simulink subsystem "PieroMMG"  (R2023b)
settings: Solver=VariableStepAuto  StartTime=0.0  StopTime=10.0  RelTol=1e-3
settings Model: Creator=jaime  LastModifiedBy=jaime

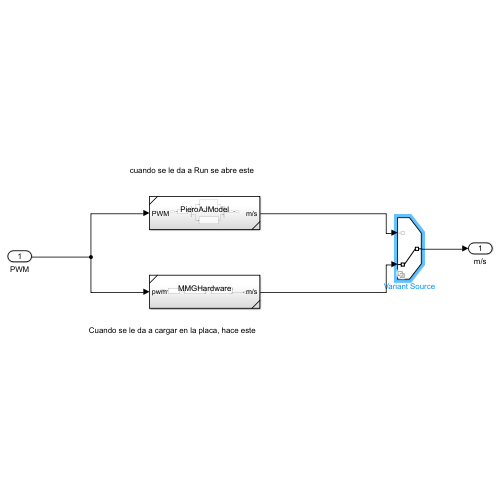
[thumbnail: Simulink's stored preview of the top-level diagram]
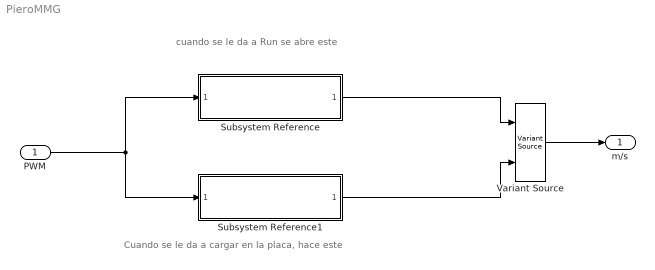
== system PieroMMG ==
  note: Cuando se le da a cargar en la placa, hace este
  note: cuando se le da a Run se abre este
  PWM : Inport
  Subsystem Reference : Subsystem  ReferencedSubsystem=PieroAJModel
  Subsystem Reference1 : Subsystem  ReferencedSubsystem=MMGHardware
  Variant Source : VariantSource  VariantControlMode=sim codegen switching
  m/s : Outport
  wires:
  Subsystem Reference1/1 -> Variant Source/2
  Subsystem Reference/1 -> Variant Source/1
  Variant Source/1 -> m/s/1
  PWM/1 -> Subsystem Reference1/1, Subsystem Reference/1
